simulink model "black_box_ex5"  (Simulink 7.1)
settings: Solver=ode45  StartTime=0.0  StopTime=40  RelTol=1e-3
undefined symbols (not defined in the file or in its folder): gcbh, xlBlockLoadCallback
libraries: xbsIndex_r4 x6, xbsCopyrightNotice_r4 x1
settings Model: Creator=alexc  LastModifiedBy=douangp  ExtModeTrigMode=oneshot  ExtModeArmWhenConnect=off
settings DataIOCC: LimitDataPoints=off  SignalLoggingName=sigsOut
settings OptimizationCC: BlockReduction=off  BooleanDataType=off  InlineInvariantSignals=on
settings DebuggingCC: SaveWithParameterizedLinksMsg=none  SignalResolutionControl=TryResolveAllWithWarning  SolverPrmCheckMsg=none  MultiTaskDSMMsg=warning  MultiTaskCondExecSysMsg=none  StrictBusMsg=None
settings HardwareCC: TargetUnknown=on
settings RTWCC: IncludeERTFirstTime=on
settings GRTTargetCC: TargetFcnLib=ansi_tfl_tmw.mat

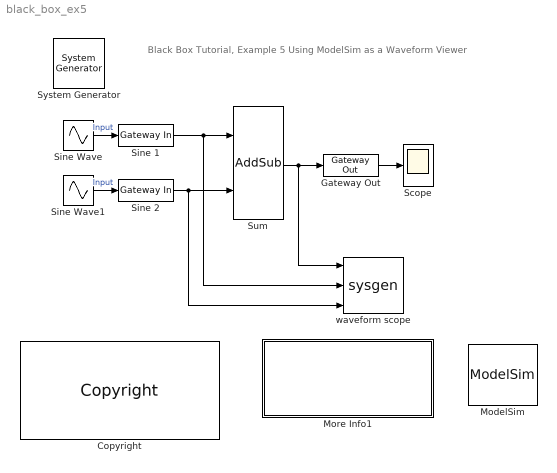
== system black_box_ex5 ==
  note: Black Box Tutorial, Example 5
      | Using ModelSim as a Waveform Viewer
  " System Generator" : xbsIndex_r4/ System Generator  Tag=genX  SystemSampleTime=-1  xilinxfamily=virtex6  part=xc6vlx240t  speed=-1  package=ff1156  synthesis_tool=XST  clock_wrapper=Clock Enables  directory=./netlist  testbench=off  simulink_period=1  sysclk_period=10  dcm_input_clock_period=100  incr_netlist=off  trim_vbits=Everywhere in SubSystem  dbl_ovrd=According to Block Masks  core_generation=According to Block Masks  run_coregen=off  deprecated_control=off  eval_field=0  block_type=sysgen
      settings: block_version=10.1.3
  Copyright : xbsCopyrightNotice_r4/Copyright  copyrighttext="Copyright (c) 2009  by  Xilinx, Inc. All rights reserved.<br><br>This file contains proprietary, confidential information of Xilinx, Inc., is distributed under licensefrom Xilinx, Inc., and may be used, copied and/or disclosed only pursuant to the terms of a valid licenseagreement with Xilinx, Inc. Xilinx hereby grants you a license to use this file solely for design,simulation, implementation and creation of design files limited to Xilinx devices or technologies. Use with non-Xilinx devices or technologies is expressly prohibited and immediately terminates your license unless covered by a separate agreement.<br><br>Xilinx is providing this design, code, or information \"as-is\" solely for use in developing programs and solutions for Xilinx devices, with no obligation on the part of Xilinx to provide support. By providingthis design, code, or information as one possible implementation of this feature, application or standard,Xilinx is making no representation that this implementation is free from any claims of infringement. Youare responsible for obtaining any rights you may require for your implementation. Xilinx expressly disclaimsany warranty whatsoever with respect to the adequacy of the implementation, including but not limited to anywarranties or representations that this implementation is free from claims of infringement, implied warrantiesof merchantability or fitness for a particular purpose.<br><br>Xilinx products are not intended for use in life support appliances, devices, or systems. Use in such applications is expressly prohibited.<br><br>Any modifications that are made to the Source Code are done at the user's sole risk and will be unsupported.<br><br>This copyright and support notice must be retained as part of this text at all times. (c) Copyright 1995-2009 Xilinx, Inc. All rights reserved."  block_type=copyright
      settings: block_version=10.1.3
      settings: infoedit=|
      | Copyright(C) 2008 by  Xilinx, Inc. All rights reserved.<br>
      | <br>
      | This file contains proprietary, confidential information of Xilinx, Inc., is distributed under license
      | from Xilinx, Inc., and may be used, copied and/or disclosed only pursuant to the terms of a valid license
      | agreement with Xilinx, Inc. Xilinx hereby grants you a license to use this file solely for design,
      | simulation, implementation and creation of design files limited to Xilinx devices or technologies. Use
      | with non-Xilinx devices or technologies is expressly prohibited and immediately terminates your license
      | unless covered by a separate agreement.<br>
      | <br>
      | Xilinx is providing this design, code, or information "as-is" solely for use in developing programs and
      | solutions for Xilinx devices, with no obligation on the part of Xilinx to provide support. By providing
      | this design, code, or information as one possible implementation of this feature, application or standard,
      | Xilinx is making no representation that this implementation is free from any claims of infringement. You
      | are responsible for obtaining any rights you may require for your implementation. Xilinx expressly disclaims
      | any warranty whatsoever with respect to the adequacy of the implementation, including but not limited to any
      | warranties or representations that this implementation is free from claims of infringement, implied warranties
      | of merchantability or fitness for a particular purpose.<br>
      | <br>
      | Xilinx products are not intended for use in life support appliances, devices, or systems. Use in such
      | applications is expressly prohibited.<br>
      | <br>
      | Any modifications that are made to the Source Code are done at the user's sole risk and will be unsupported.<br>
      | <br>
      | This copyright and support notice must be retained as part of this text at all times.
      | (c) Copyright 1995-2008 Xilinx, Inc. All rights reserved.
  Gateway Out : xbsIndex_r4/Gateway Out  hdl_port=on  timing_constraint=None  locs_specified=off  LOCs={}  block_type=gatewayout
      settings: infoedit="Gateway out block.  Converts Xilinx fixed point inputs into ouputs of type Simulink integer, double, or fixed point.<P><P>Hardware notes:  In hardware these blocks become top level output ports or are discarded, depending on how they are configured."  xl_area=[0, 0, 0, 0, 0, 0, 0]  block_version=VER_STRING_GOES_HERE
  ModelSim : xbsIndex_r4/ModelSim  dir=./modelsim  waveform=on  leave_open=on  skip_compile=off  use_unisim=off  custom_scripts=on  post_vsim_script=waveform.do  startup_timeout=40  block_type=hdlcosim
      settings: infoedit="Allow other blocks to schedule HDL co-simulation tasks.<P><P>Note that selecting \"Skip compilation\" when inappropriate can cause simulation errors and failures. Please refer to the block help for details."  block_version=VER_STRING_GOES_HERE
  More Info1 : Subsystem
      settings: OpenFcn=xlDoc('-book','sysgen', '-title', 'Black Box');
      mask Display: disp('Double click\n for System Generator\n documentation on\n related topics.')
  Scope : Scope
      settings: YMin=-1  YMax=2
  Sine 1 : xbsIndex_r4/Gateway In  arith_type="Signed  (2's comp)"  n_bits=8  bin_pt=6  quantization="Round  (unbiased: +/- Inf)"  overflow=Saturate  period=1  dbl_ovrd=off  timing_constraint=None  locs_specified=off  LOCs={}  block_type=gatewayin
      settings: infoedit="Gateway in block.  Converts inputs of type Simulink integer, double and fixed point to  Xilinx fixed point type.<P><P>Hardware notes:  In hardware these blocks become top level input ports."  xl_area=[0, 0, 0, 0, 0, 0, 0]  block_version=VER_STRING_GOES_HERE
  Sine 2 : xbsIndex_r4/Gateway In  arith_type="Signed  (2's comp)"  n_bits=8  bin_pt=6  quantization="Round  (unbiased: +/- Inf)"  overflow=Saturate  period=1  dbl_ovrd=off  timing_constraint=None  locs_specified=off  LOCs={}  block_type=gatewayin
      settings: infoedit="Gateway in block.  Converts inputs of type Simulink integer, double and fixed point to  Xilinx fixed point type.<P><P>Hardware notes:  In hardware these blocks become top level input ports."  xl_area=[0, 0, 0, 0, 0, 0, 0]  block_version=VER_STRING_GOES_HERE
  Sine Wave : Sin  Amplitude=.5  Frequency=2*pi/23  Phase=pi/6  SampleTime=1
  Sine Wave1 : Sin  Amplitude=0.75  Frequency=2*pi/13  SampleTime=1
  Sum : xbsIndex_r4/AddSub  mode=Addition  use_carryin=off  use_carryout=off  en=off  latency=1  precision=Full  arith_type=Unsigned  n_bits=8  bin_pt=2  quantization=Truncate  overflow=Wrap  dbl_ovrd=off  use_behavioral_HDL=off  hw_selection=Fabric  pipelined=off  use_rpm=off  block_type=addsub
      settings: xl_area=[0, 0, 0, 0, 0, 0, 0]  block_version=VER_STRING_GOES_HERE
  waveform scope : S-Function  LoadFcn=xlBlockLoadCallback(gcbh);  FunctionName=sysgen  Parameters=ptable_  EnableBusSupport=off  mask(Xilinx Blackbox Scope Example){infoedit=Incorporates black box HDL and simulation model into a System Generator design.<P><P>You must supply a Black Box with certain information about the HDL component you would like to bring into System Generator. This information is provided through a Matlab function.<P><P>When "Simulation Mode" is set to "Inactive", you will typically want to provide a separate simulation model by using a Simulation Multiplexer.<P>When "Simulation Mode" is set to "External co-simulator", you must include a ModelSim block in the design., nports=3, init_code=scope_config, sim_method=External co-simulator, sim_method_sgadvanced=, engine_block=ModelSim, xl_use_area=off, xl_use_area_sgadvanced=, xl_area=[0,0,0,0,0,0,0], block_version=VER_STRING_GOES_HERE, has_advanced_control=0, sggui_pos=-1,-1,-1,-1, block_type=blackbox2, sg_icon_stat=60,56,3,0,white,blue,0,1b2bc80a,right,, sg_mask_display=|, sg_list_contents=}
      mask sg_mask_display=|
      | fprintf('','COMMENT: begin icon graphics ');
      | patch([0 1 1 0 ],[0 0 1 1 ],[0.77 0.82 0.91]);
      | patch([0.25 0.1 0.316667 0.1 0.25 0.5 0.566667 0.633333 0.9 0.683333 0.483333 0.333333 0.533333 0.333333 0.483333 0.683333 0.9 0.633333 0.566667 0.5 0.25 ],[0.107143 0.267857 0.5 0.732143 0.892857 0.892857 0.821429 0.892857 0.892857 0.660714 0.875 0.714286 0.5 0.285714 0.125 0.339286 0.107143 0.107143 0.178571 0.107143 0.107143 ],[0.98 0.96 0.92]);
      | plot([0 1 1 0 0 ],[0 0 1 1 0 ]);
      | fprintf('','COMMENT: end icon graphics');
      |
      | fprintf('','COMMENT: begin icon text ');
      | color('black');port_label('input',1,'sig1');
      | color('black');port_label('input',2,'sig2');
      | color('black');port_label('input',3,'sig3');
      | fprintf('','COMMENT: end icon text');
      | fprintf('','COMMENT: Make no changes above this line -- machine generated code. ');
      mask prompts: infoedit ""; nports "Number of input ports"; init_code "Block configuration m-function"; sim_method "Simulation mode"; engine_block "HDL co-simulator to use  (specify helper block by name)"; xl_use_area "Define FPGA area for resource estimation"; xl_area "FPGA area [slices, FFs, BRAMs, LUTs, IOBs, emb. mults, TBUFs]"; block_version ""; has_advanced_control ""; sggui_pos ""; block_type ""; sg_icon_stat ""; sg_mask_display ""; sg_list_contents ""
      mask init:
      | xlMungeMaskParams;
      | 
      | mdlPath = xlGetMdlDir(bdroot);
      | 
      | refBlk = get_param(gcb,'referenceBlock');
      | if (isempty(refBlk) | strncmp(refBlk,'xbsIndex',8))
      | srcPath = mdlPath;
      | else
      | srcPath = xlPathToReference;
      | if (isempty(srcPath))
      | srcPath = mdlPath;
      | end
      | end
      | 
      | if (sim_method==3)
      | validEngineBlock = 0;
      | try
      | engineBlock = xlBlockNameRelPath(get_param(gcb,'Parent'),engine_block);
      | catch
      | engineBlock = '//';
      | end
      | try 
      | engineWorkDir = get_param(engineBlock,'dir');
      | validEngineBlock = 1;
      | engine_handle = get_param(engineBlock,'Handle');
      | catch
      | end
      | end
      | 
      | % build black box config function
      | block_config = ['sysgen_blockset:black_box_config:' init_code];
      | 
      | serialized_declarations = '{''engine_handle''=>''Double'',''sim_method''=>''Int'',''validEngineBlock''=>''Int'',''engineWorkDir''=>''String'',''engine_block''=>''String'',''init_code''=>''String'',''mdlPath''=>''String'',''srcPath''=>''String'',''block_config''=>''String'',}';
      | ptable_ = xlblockprep(get_param(gcb, 'MaskWSVariables'));
      settings: CopyFcn=xlBlockMoveCallback(gcbh);xlbbCopyCallback;  DeleteFcn=xlDestroyGui(gcbh);  ModelCloseFcn=xlDestroyGui(gcbh);  PreSaveFcn=xlBlockPreSaveCallback(gcbh);  PostSaveFcn=xlBlockPostSaveCallback(gcbh);  DestroyFcn=xlDestroyGui(gcbh);  MoveFcn=xlBlockMoveCallback(gcbh);
      mask Help: xlWeb(xlhtmldoclink('Black Box'));
      mask StyleString: edit,popup(1|2|3|4),edit,popup(Inactive|ISE Simulator|External co-simulator),edit,edit,checkbox,edit,edit,edit,edit,edit,edit,edit,edit,edit
      mask Display:
      | fprintf('','COMMENT: begin icon graphics ');
      | patch([0 1 1 0 ],[0 0 1 1 ],[0.77 0.82 0.91]);
      | patch([0.25 0.1 0.316667 0.1 0.25 0.5 0.566667 0.633333 0.9 0.683333 0.483333 0.333333 0.533333 0.333333 0.483333 0.683333 0.9 0.633333 0.566667 0.5 0.25 ],[0.107143 0.267857 0.5 0.732143 0.892857 0.892857 0.821429 0.892857 0.892857 0.660714 0.875 0.714286 0.5 0.285714 0.125 0.339286 0.107143 0.107143 0.178571 0.107143 0.107143 ],[0.98 0.96 0.92]);
      | plot([0 1 1 0 0 ],[0 0 1 1 0 ]);
      | fprintf('','COMMENT: end icon graphics');
      | 
      | fprintf('','COMMENT: begin icon text ');
      | color('black');port_label('input',1,'sig1');
      | color('black');port_label('input',2,'sig2');
      | color('black');port_label('input',3,'sig3');
      | fprintf('','COMMENT: end icon text');
      | fprintf('','COMMENT: Make no changes above this line -- machine generated code. ');
  wires:
  Gateway Out/1 -> Scope/1
  Sine Wave/1 -> Sine 1/1  "Input"
  Sine Wave1/1 -> Sine 2/1  "Input"
  Sine 2/1 -> Sum/2, waveform scope/3
  Sum/1 -> Gateway Out/1, waveform scope/1
  Sine 1/1 -> Sum/1, waveform scope/2

== system black_box_ex5/More Info1 ==
